simulink library "HeatPump"  (Simulink 8.2)
settings: Solver=ode45  StartTime=0.0  StopTime=10.0  RelTol=1e-3
undefined symbols (not defined in the file): THBout_cold, THBout_hot
libraries: carnot x3
settings Model: Creator=lena.frank  LastModifiedBy=drhf

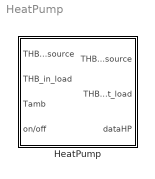
== system HeatPump ==
  HeatPump : Subsystem  mask(heat pump){Tcin=[-5 15], Thout=[35 45 55 60], Qdotc=[14000 12500 10000 9200;26900 24000 21700 20000], Qdoth=[18000 17200 16500 16000;31500 29500 27800 27000], Pel=[4400 5500 7000 7500;4600 6000 7000 7500], caph=80000, capc=50000, UA=7, linc=10, quac=10, linh=10, quah=10}
      mask prompts: Tcin "inlet source temperature vector (°C)"; Thout "outlet load temperature vector (°C)"; Qdotc "source power matrix (W)"; Qdoth "heating power matrix (W)"; Pel "electric power matrix (W)"; caph "thermal capacity hot loop [J/K]"; capc "thermal capacity cold loop [J/K]"; UA "heat loss coefficient [W/K]"; linc "Cold side linear massflow dependant pressure drop in [Pa*s/kg]"; quac "Cold side quadratic massflow dependant pressure drop hot side in [Pa*s²/kg]"; linh "Hot side linear massflow dependant pressure drop in [Pa*s/kg]"; quah "Hot side quadratic massflow dependant pressure drop hot side in [Pa*s²/kg]"
      mask help:
      | Linearized heat pump model. Uses measured data according to EN 14511 as input.
      | heating power: Qdot_h = K1*Tcold_in + K2*Thot_out + K3
      | electric power: Pel = K4*Tcold_in + K5*Thot_out + K6
      | source power: Qdot_c = -K7*Tcold_in - K8*Thot_out - K9
      | differential equation: cap*dTh/dt = Qdot + mdot*cp*(T_in-T) + UA*(Tamb-T)
      | with: cap = mass * heat_capactiy
      | See hp_param.m for the parameters K1 to K9.
      | Literature: Schwamberger, K.: Fortschrittsberichete VDI, Nr. 263, 1991
      mask init:
      | % Matrix construction for hp_param
      | A = reshape(Qdoth',numel(Qdoth),1);
      | A = [A reshape(Qdotc',numel(Qdotc),1)];
      | A = [A reshape(Pel',numel(Pel),1)];
      | Thout_temp = [];
      | Tcin_temp = [];
      | for i=1:numel(Tcin)
      |     for j=1:numel(Thout)
      |         Tcin_temp = [Tcin_temp ; Tcin(i)];
      |     end
      |     Thout_temp = [Thout_temp ; Thout'];
      | end
      | A = [A Tcin_temp Thout_temp];
      | 
      | K = hp_param(A);
      | caph = max(1,caph);
      | capc = max(1,capc);
      mask Help: web(fullfile(path_carnot('help'),'heatpump.html'),'-helpbrowser')
      mask Display:
      | plot(-20,-10,120,110,[10,20,40,60,80,90,90,80,60,40,20,10,10],[60,80,90,90,80,60,40,20,10,10,20,40,60],[40,20],[90,20],[60,80],[90,20],[50,50],[30,50],[60,40],[40,40],[57,43],[33,46],[44,57],[34,46])
      | port_label('input',1,'THB_c')
      | port_label('input',2,'THB_h')
      | port_label('input',3,'Ta')
      | port_label('input',4,'ctr')
      | port_label('output',1,'THB_c')
      | port_label('output',2,'THB_h')
      | port_label('output',3,'HPdat')

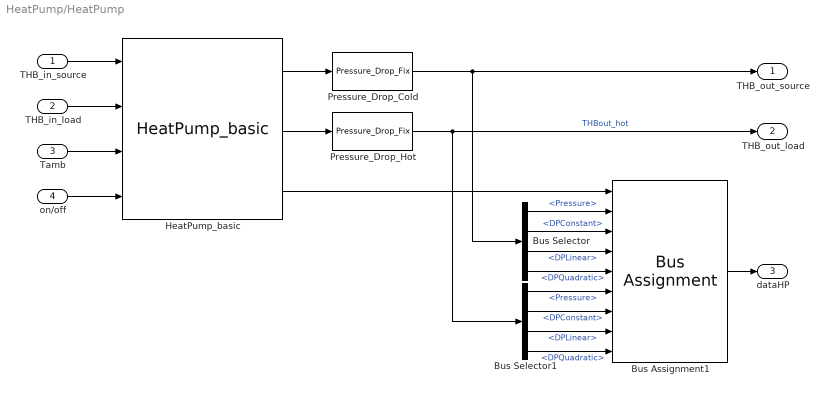
== system HeatPump/HeatPump ==
  THB_in_source : Inport
  THB_in_load : Inport  Port=2
  Tamb : Inport  Port=3
  on/off : Inport  Port=4
  Bus Assignment1 : BusAssignment  AssignedSignals=THBout_cold.Pressure,THBout_cold.DPConstant,THBout_cold.DPLinear,THBout_cold.DPQuadratic,THBout_hot.Pressure,THBout_hot.DPConstant,THBout_hot.DPLinear,THBout_hot.DPQuadratic
  Bus Selector : BusSelector  OutputSignals=Pressure,DPConstant,DPLinear,DPQuadratic
  Bus Selector1 : BusSelector  OutputSignals=Pressure,DPConstant,DPLinear,DPQuadratic
  HeatPump_basic : carnot/Basic/Thermal_Models/HeatPump_basic  K=K  caph=caph  capc=capc  UA=UA
  Pressure_Drop_Cold : carnot/Basic/Pressure_Drop/Pressure_Drop_Fix  con=0  lin=linc  qua=quac
  Pressure_Drop_Hot : carnot/Basic/Pressure_Drop/Pressure_Drop_Fix  con=0  lin=linh  qua=quah
  THB_out_source : Outport
  THB_out_load : Outport  Port=2
  dataHP : Outport  Port=3
  wires:
  Pressure_Drop_Hot/1 -> THB_out_load/1, Bus Selector1/1  "THBout_hot"
  HeatPump_basic/2 -> Pressure_Drop_Hot/1
  THB_in_source/1 -> HeatPump_basic/1
  THB_in_load/1 -> HeatPump_basic/2
  Tamb/1 -> HeatPump_basic/3
  on/off/1 -> HeatPump_basic/4
  HeatPump_basic/1 -> Pressure_Drop_Cold/1
  Pressure_Drop_Cold/1 -> THB_out_source/1, Bus Selector/1
  HeatPump_basic/3 -> Bus Assignment1/1
  Bus Assignment1/1 -> dataHP/1
  Bus Selector/1 -> Bus Assignment1/2  "<Pressure>"
  Bus Selector/2 -> Bus Assignment1/3  "<DPConstant>"
  Bus Selector/3 -> Bus Assignment1/4  "<DPLinear>"
  Bus Selector/4 -> Bus Assignment1/5  "<DPQuadratic>"
  Bus Selector1/1 -> Bus Assignment1/6  "<Pressure>"
  Bus Selector1/2 -> Bus Assignment1/7  "<DPConstant>"
  Bus Selector1/3 -> Bus Assignment1/8  "<DPLinear>"
  Bus Selector1/4 -> Bus Assignment1/9  "<DPQuadratic>"
